simulink model "simulation_darko_complet_fuel_op"  (R2020b)
settings: Solver=VariableStepAuto  StartTime=0.0  StopTime=20  RelTol=1e-3
values from neighbouring files (symbols this model uses):
  controlleur = generateContolleur(drone)    [run_darko_droit_complet_fuel_op.m]
  drone = struct('MASS',               0.492,                      'INERTIA',            eye(3),                     'G',                  9.81,                       'P_P1_CG',            [1; 1; 1],                  'P_P2_CG',            [1; 1; 1],                  'P_A1_CG',            [1; 1; 1],                  'P_A2_CG',            [1; 1; 1],                  'INERTIA_PROP_X',     5.1116e-6,            ...(+959 chars)    [generateDarko.m]    (also in run_darko_droit_complet_fuel_op.m = generateDarko())
  f_initial = drone.MASS*drone.G    [run_darko_droit_complet_fuel_op.m]
  initial_state = [p_initial; v_initial; omega_initial; q_initial]    [run_darko_droit_complet_fuel_op.m]
  position_cible = 1*[1; 1; 1]    [run_darko_droit_complet_fuel_op.m]
  q_d_initial = ToQuaternion(yaw_d, pitch_d, roll_d)    [run_darko_droit_complet_fuel_op.m]
libraries: simulink_extras x3, sharedtransform x1
settings Model: Creator=florian  LastModifiedBy=florian

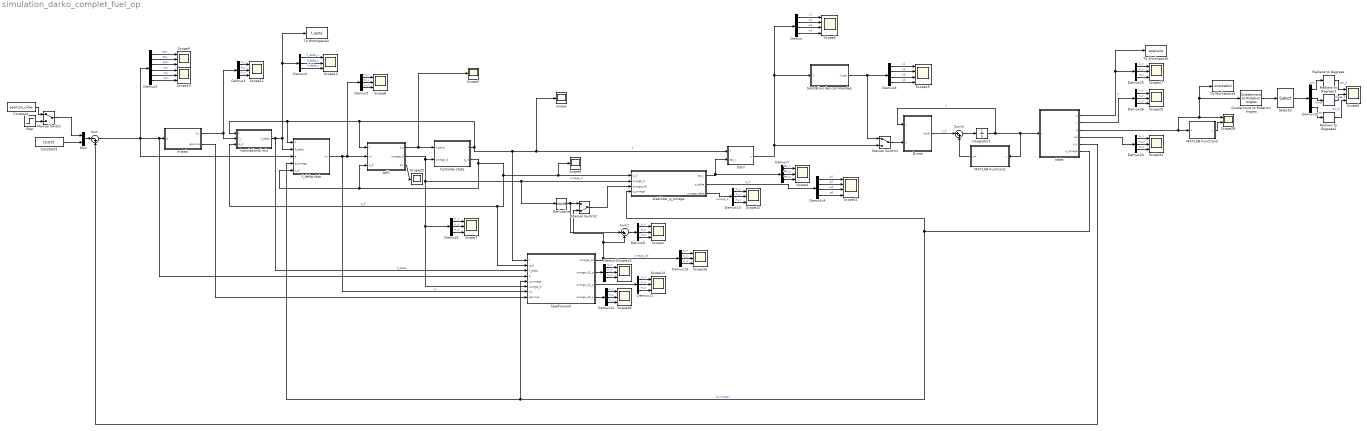
== system simulation_darko_complet_fuel_op ==
  Constant : Constant  Value=position_cible
  Constant1 : Constant  Value=[0;0;0]
  Contoller state : Subsystem
  Demux : Demux
  Demux{1,3..7,9..13,15,24..26} (15 alike) : Demux  Outputs=3
  Demux14 : Demux
  Demux2 : Demux  Outputs=6
  Demux8 : Demux
  Derivative : Derivative  CoefficientInTFapproximation=1/1000
  Drone : MATLAB Function  TreatAsAtomicUnit=on
  Integrator1 : Integrator  InitialCondition=initial_state
  MATLAB Function2 : MATLAB Function  TreatAsAtomicUnit=on
  MATLAB Function3 : MATLAB Function  TreatAsAtomicUnit=on
  Manual Switch : ManualSwitch
  Manual Switch1 : ManualSwitch
  Manual Switch2 : ManualSwitch  CurrentSetting=0
  Mux : Mux  Inputs=2
  Quaternions to Rotation Angles : sharedtransform/Quaternions to Rotation Angles  rotationOrder=ZXY  aMode=aMode
      settings: SourceProductBaseCode=AE,PW,MT,UV,VE,VP
  Radians to Degrees : simulink_extras/Transformations/Radians to Degrees
  Radians to Degrees1 : simulink_extras/Transformations/Radians to Degrees
  Radians to Degrees2 : simulink_extras/Transformations/Radians to Degrees
  Satutation des commandes : Subsystem
  Scope{,2,6,20} (4 alike) : Scope
  Scope{1,3..4,7..14,16,18,22,27,29,34} (17 alike) : Scope  NumInputPorts=3
  Scope15 : Scope  NumInputPorts=4
  Scope21 : Scope  NumInputPorts=4
  Scope28 : Scope  NumInputPorts=2
  Scope5 : Scope  NumInputPorts=4
  Selector : Selector  InputPortWidth=3  IndexOptions=Index vector (dialog)  Indices=[2 3 1]  OutputSizes=1
  Step : Step  Time=10  Before=position_cible  After=[0;0;0]  SampleTime=0
  Sum : Sum  Inputs=|-+
  Sum1 : Sum  Inputs=|+-
  Sum5 : Sum  Inputs=|++
  To Workspace1 : ToWorkspace  VariableName=positions  SampleTime=-1
  To Workspace2 : ToWorkspace  VariableName=f_delta  SampleTime=-1
  To Workspace3 : ToWorkspace  VariableName=orientation  SampleTime=-1
  distri : MATLAB Function  TreatAsAtomicUnit=on
  e stab : MATLAB Function  TreatAsAtomicUnit=on
  f_delta stab : MATLAB Function  TreatAsAtomicUnit=on
  feedforward : MATLAB Function  TreatAsAtomicUnit=on
  split : MATLAB Function  TreatAsAtomicUnit=on
  stabilizer_q_omega : MATLAB Function  TreatAsAtomicUnit=on
  state : MATLAB Function  TreatAsAtomicUnit=on
  translational mis : MATLAB Function  TreatAsAtomicUnit=on
  wires:
  Manual Switch/1 -> Mux/1
  Mux/1 -> Sum/1
  f_delta stab/1(nu) -> feedforward/7(nu), Demux5/1, split/2(nu)  "nu"
  Demux4/2 -> Scope12/2  "f_delta_y"
  Contoller state/2(q_d) -> f_delta stab/5(q_d), split/3(q_d), feedforward/2(q_d), translational mis/3(q_d), Scope6/1, stabilizer_q_omega/1(q_d)  "q_d"
  Step/1 -> Manual Switch/2
  Demux9/2 -> Scope7/2  "w_y"
  Demux2/4 -> Scope10/1  "vpx"
  stabilizer_q_omega/3(omega_delta) -> Demux15/1  "omega_d"
  Demux15/3 -> Scope22/3  "w_z"
  split/2(omega_d) -> feedforward/6(omega_d), Demux9/1, Derivative/1, stabilizer_q_omega/2(omega_d), Contoller state/2(omega_d)  "omega_d"
  translational mis/1(f_delta) -> feedforward/3(f_delta), Demux4/1, To Workspace2/1, f_delta stab/2(f_delta)  "f_delta"
  Demux15/1 -> Scope22/1  "w_x"
  Demux15/2 -> Scope22/2  "w_y"
  Demux2/1 -> Scope9/1  "epx"
  Demux2/5 -> Scope10/2  "vpy"
  Constant/1 -> Manual Switch/1
  Demux3/3 -> Scope11/3  "fr_z"
  Demux4/3 -> Scope12/3  "f_delta_z"
  Constant1/1 -> Mux/2
  Demux5/1 -> Scope8/1  "nu_x"
  Demux4/1 -> Scope12/1  "f_delta_x"
  stabilizer_q_omega/1(tau_r) -> Demux7/1, distri/2(tau_r)
  split/1(f_d) -> Scope2/1, Contoller state/1(f_point)
  Demux5/3 -> Scope8/3  "nu_z"
  Demux9/3 -> Scope7/3  "w_z"
  split/3(err) -> Scope20/1
  Demux3/1 -> Scope11/1  "fr_x"
  Contoller state/1(f) -> f_delta stab/1(f), translational mis/1(f), split/1(f), feedforward/1(f), Scope/1, distri/1(f)  "f"
  Demux2/6 -> Scope10/3  "vpz"
  Demux3/2 -> Scope11/2  "fr_y"
  Demux2/2 -> Scope9/2  "epy"
  Demux9/1 -> Scope7/1  "w_x"
  Demux2/3 -> Scope9/3  "epz"
  Demux5/2 -> Scope8/2  "nu_y"
  e stab/1(f_r) -> translational mis/2(f_r), Demux3/1
  Sum/1 -> feedforward/4(e), e stab/1(e), f_delta stab/3(e), Demux2/1
  Manual Switch2/1 -> stabilizer_q_omega/3(omega_dd)
  Derivative/1 -> Sum1/1, Manual Switch2/1
  feedforward/1(omega_dd) -> Demux13/1, Sum1/2, Manual Switch2/2  "omega_dd"
  Demux1/3 -> Scope13/3  "w_z"
  feedforward/4(omega_d3_p) -> Demux12/1
  Demux11/2 -> Scope14/2  "w_y"
  Demux12/3 -> Scope18/3  "w_z"
  feedforward/2(omega_d1_p) -> Demux1/1
  Demux12/1 -> Scope18/1  "w_x"
  Demux11/1 -> Scope14/1  "w_x"
  Demux1/2 -> Scope13/2  "w_y"
  Demux11/3 -> Scope14/3  "w_z"
  Demux12/2 -> Scope18/2  "w_y"
  feedforward/3(omega_d2_p) -> Demux11/1
  Demux1/1 -> Scope13/1  "w_x"
  e stab/2(gamma) -> feedforward/8(gamma)
  Demux7/2 -> Scope4/2  "tau_y"
  Satutation des commandes/1(U_sat) -> Manual Switch1/1, Demux8/1
  state/2(v) -> Demux26/1
  Demux25/1 -> Scope27/1  "p_x"
  Demux26/1 -> Scope29/1  "v_x"
  Integrator1/1 -> Drone/1(x), MATLAB Function2/1(x), state/1(x)  "x"
  state/1(p) -> To Workspace1/1, Demux25/1  "p"
  Demux/1 -> Scope5/1  "u1"
  distri/1(u) -> Satutation des commandes/1(U), Demux/1, Manual Switch1/2
  Sum5/1 -> Integrator1/1
  state/3(q) -> Scope28/1, To Workspace3/1, Quaternions to Rotation Angles/1, MATLAB Function3/1(u)
  Demux24/1 -> Scope34/1  "w_x"
  Demux25/2 -> Scope27/2  "p_y"
  Demux7/3 -> Scope4/3  "tau_z"
  Demux/2 -> Scope5/2  "u2"
  stabilizer_q_omega/2(q_delta) -> Demux14/1  "q_d"
  Drone/1(dxdt) -> Sum5/1  "x_d"
  Demux8/2 -> Scope15/2  "u2"
  MATLAB Function3/1(y) -> Scope28/2
  Demux7/1 -> Scope4/1  "tau_x"
  Demux14/3 -> Scope21/3  "q3"
  state/6(q_omega) -> stabilizer_q_omega/4(q_omega), feedforward/5(q_omega), f_delta stab/4(q_omega)  "(q,omega)"
  Demux25/3 -> Scope27/3  "p_z"
  MATLAB Function2/1(cor) -> Sum5/2
  Manual Switch1/1 -> Drone/2(u)
  Demux14/4 -> Scope21/4  "q4"
  Demux26/3 -> Scope29/3  "v_z"
  Demux8/4 -> Scope15/4  "u4"
  Demux8/1 -> Scope15/1  "u1"
  Demux14/1 -> Scope21/1  "q1"
  Demux/4 -> Scope5/4  "u4"
  Demux24/3 -> Scope34/3  "w_z"
  Demux14/2 -> Scope21/2  "q2"
  Demux8/3 -> Scope15/3  "u3"
  state/5(p_v) -> Sum/2
  state/4(wb) -> Demux24/1
  Demux/3 -> Scope5/3  "u3"
  Demux24/2 -> Scope34/2  "w_y"
  Demux26/2 -> Scope29/2  "v_y"
  Quaternions to Rotation Angles/1 -> Selector/1
  Radians to Degrees1/1 -> Scope3/2  "theta_d"
  Demux10/1 -> Radians to Degrees/1  "phi"
  Demux10/3 -> Radians to Degrees2/1  "psi"
  Selector/1 -> Demux10/1
  Radians to Degrees/1 -> Scope3/1  "phi_d"
  Demux10/2 -> Radians to Degrees1/1  "theta"
  Radians to Degrees2/1 -> Scope3/3  "psi_d"
  Sum1/1 -> Demux6/1
  Demux6/1 -> Scope1/1  "w_x"
  Demux6/3 -> Scope1/3  "w_z"
  Demux6/2 -> Scope1/2  "w_y"
  Demux13/1 -> Scope16/1  "w_x"
  Demux13/3 -> Scope16/3  "w_z"
  Demux13/2 -> Scope16/2  "w_y"

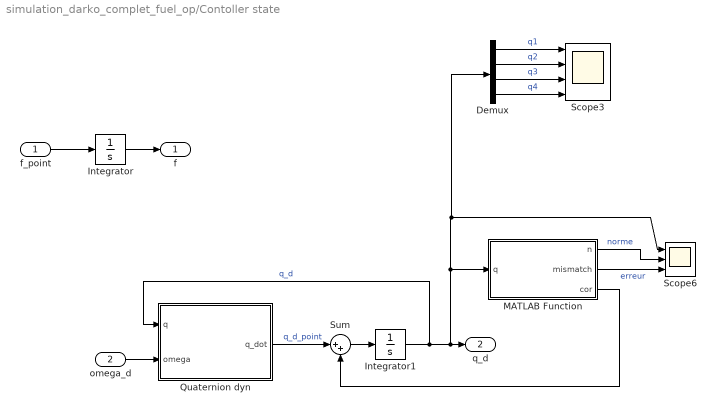
== system simulation_darko_complet_fuel_op/Contoller state ==
  f_point : Inport
  omega_d : Inport  Port=2
  Demux : Demux
  Integrator : Integrator  InitialCondition=f_initial
  Integrator1 : Integrator  InitialCondition=q_d_initial
  MATLAB Function : MATLAB Function  TreatAsAtomicUnit=on
  Quaternion dyn : MATLAB Function  TreatAsAtomicUnit=on
  Scope3 : Scope  NumInputPorts=4
  Scope6 : Scope  NumInputPorts=3
  Sum : Sum  Inputs=|++
  f : Outport
  q_d : Outport  Port=2
  wires:
  Integrator/1 -> f/1
  f_point/1 -> Integrator/1
  Integrator1/1 -> Quaternion dyn/1(q), Demux/1, Scope6/1, MATLAB Function/1(q), q_d/1  "q_d"
  omega_d/1 -> Quaternion dyn/2(omega)
  Quaternion dyn/1(q_dot) -> Sum/1  "q_d_point"
  Sum/1 -> Integrator1/1
  MATLAB Function/3(cor) -> Sum/2
  MATLAB Function/1(n) -> Scope6/2  "norme"
  MATLAB Function/2(mismatch) -> Scope6/3  "erreur"
  Demux/3 -> Scope3/3  "q3"
  Demux/2 -> Scope3/2  "q2"
  Demux/1 -> Scope3/1  "q1"
  Demux/4 -> Scope3/4  "q4"

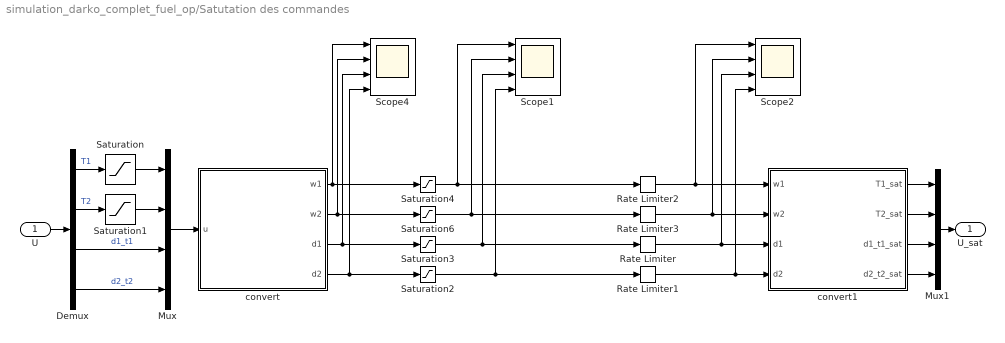
== system simulation_darko_complet_fuel_op/Satutation des commandes ==
  U : Inport
  Demux : Demux
  Mux : Mux
  Mux1 : Mux
  Rate Limiter : RateLimiter  RisingSlewLimit=drone.ELEVON_RATE_CHANGE  FallingSlewLimit=-drone.ELEVON_RATE_CHANGE  SampleTimeMode=inherited
  Rate Limiter1 : RateLimiter  RisingSlewLimit=drone.ELEVON_RATE_CHANGE  FallingSlewLimit=-drone.ELEVON_RATE_CHANGE  SampleTimeMode=inherited
  Rate Limiter2 : RateLimiter  RisingSlewLimit=drone.MOTOR_RATE_CHANGE  FallingSlewLimit=-drone.MOTOR_RATE_CHANGE  SampleTimeMode=inherited
  Rate Limiter3 : RateLimiter  RisingSlewLimit=drone.MOTOR_RATE_CHANGE  FallingSlewLimit=-drone.MOTOR_RATE_CHANGE  SampleTimeMode=inherited
  Saturation : Saturate  UpperLimit=100  LowerLimit=0.001
  Saturation1 : Saturate  UpperLimit=100  LowerLimit=0.001
  Saturation2 : Saturate  UpperLimit=30*(pi/180)  LowerLimit=-30*(pi/180)
  Saturation3 : Saturate  UpperLimit=30*(pi/180)  LowerLimit=-30*(pi/180)
  Saturation4 : Saturate  UpperLimit=1000  LowerLimit=200
  Saturation6 : Saturate  UpperLimit=1000  LowerLimit=200
  Scope1 : Scope  NumInputPorts=4
  Scope2 : Scope  NumInputPorts=4
  Scope4 : Scope  NumInputPorts=4
  convert : MATLAB Function  TreatAsAtomicUnit=on
  convert1 : MATLAB Function  TreatAsAtomicUnit=on
  U_sat : Outport
  wires:
  U/1 -> Demux/1
  Demux/4 -> Mux/4  "d2_t2"
  Demux/1 -> Saturation/1  "T1"
  Demux/3 -> Mux/3  "d1_t1"
  Demux/2 -> Saturation1/1  "T2"
  Saturation/1 -> Mux/1
  Mux/1 -> convert/1(u)
  convert/1(w1) -> Saturation4/1, Scope4/1
  Saturation3/1 -> Rate Limiter/1, Scope1/3
  convert/2(w2) -> Scope4/2, Saturation6/1
  convert/3(d1) -> Scope4/3, Saturation3/1
  convert/4(d2) -> Saturation2/1, Scope4/4
  convert1/1(T1_sat) -> Mux1/1
  convert1/4(d2_t2_sat) -> Mux1/4
  Mux1/1 -> U_sat/1
  Saturation1/1 -> Mux/2
  convert1/2(T2_sat) -> Mux1/2
  convert1/3(d1_t1_sat) -> Mux1/3
  Saturation2/1 -> Rate Limiter1/1, Scope1/4
  Rate Limiter/1 -> Scope2/3, convert1/3(d1)
  Saturation6/1 -> Rate Limiter3/1, Scope1/2
  Saturation4/1 -> Rate Limiter2/1, Scope1/1
  Rate Limiter1/1 -> Scope2/4, convert1/4(d2)
  Rate Limiter2/1 -> Scope2/1, convert1/1(w1)
  Rate Limiter3/1 -> Scope2/2, convert1/2(w2)

== matlab function simulation_darko_complet_fuel_op/feedforward ==
  data: f input; omega_dd output; q_d input; f_delta input; e input; q_omega input; omega_d input; nu input; gamma input; controlleur parameter; drone parameter; omega_d1_p output; omega_d2_p output; omega_d3_p output
function [omega_dd, omega_d1_p, omega_d2_p, omega_d3_p]  = feedforward(f, q_d, f_delta, e, q_omega, omega_d, nu, gamma, controlleur, drone)
%#codegen

d_etoile = controlleur.d_etoile;
kpp = controlleur.kpp;
kpd = controlleur.kpd;
k_delta = controlleur.k_delta;
m = drone.MASS;

a = controlleur.a;
b = controlleur.b;
c = controlleur.c;

ep = e(1:3);
ev = e(4:6);

q = q_omega(1:4);
omega = q_omega(5:7);

R = q2dcm(q);
Rd = q2dcm(q_d);

omega_d1_p = -(1/(f^2)) * skew_sym(d_etoile) * Rd' * nu * ( Rd * d_etoile)' * nu;
omega_d2_p = -(1/(f))* skew_sym(d_etoile) * skew_sym(omega_d) * Rd' * nu;

% ev_dot = 1/m*((R-Rd)*d_etoile*f - gamma + f_delta);
% 
% u = kpp*(ep + ev.*sqrt((abs(ev)/(2*a)).^2 + (kpd/kpp)^2));
% u_dot = kpp*(ev + ev_dot .* sqrt((abs(ev)/(2*a)).^2 + (kpd/kpp)^2) + ev .* abs(ev)./(2*a*sqrt((abs(ev)/(2*a)).^2 + (kpd/kpp)^2)));
% 
% gamma_dot = 2*a*b*c*u_dot.*exp(-c*u).*exp(-b*exp(-c*u));
% f_delta_dot = nu - gamma_dot;
% 
% term_1 = (kpp*kpd/m)*ev;
% term_2 = (kpd^2/m^2 - kpp/m) * ev_dot;
% term_3 = -(kpd/m + k_delta)*f_delta_dot;
% 
% omega_d3_p = (1/f) * skew_sym(d_etoile) * Rd'* (term_1 + term_2 + term_3); 

Gain = (kpd^2/m^2 - kpp/m);

ep_term = - Gain*kpp*ep;
ev_term = (kpp*kpd/m - Gain*kpd)*ev;
f_delta_term = (Gain + (kpd/m + k_delta)*k_delta)*f_delta;
f_term = (Gain*(R-Rd) + kpd/m * (Rd*skew_sym(omega_d) - R*skew_sym(omega)))*d_etoile* f;
nu_term = kpd/m * (Rd-R) * d_etoile * (Rd*d_etoile)'* nu;

omega_d3_p = (1/f) * skew_sym(d_etoile) * Rd'* (ep_term + ev_term + f_delta_term + f_term + nu_term); 


omega_dd = omega_d1_p + omega_d2_p + omega_d3_p ; %

== matlab function simulation_darko_complet_fuel_op/Contoller state/MATLAB Function ==
  data: n output; q input; mismatch output; cor output
function [n, mismatch, cor] = fcn(q)
%#codegen
n = norm(q);
mismatch = 1-norm(q);
cor = mismatch*q;

== matlab function simulation_darko_complet_fuel_op/Satutation des commandes/convert ==
  data: u input; w1 output; drone parameter; w2 output; d1 output; d2 output
function [w1, w2, d1, d2] = convert(u, drone)
%#codegen
kf = drone.PROP_KP;

T1 = max(u(1), 0);
T2 = max(u(2), 0);
% T1 = u(1);
% T2 = u(2);

d1_T1 = u(3);
d2_T2 = u(4);

w1 = sqrt(T1/kf);
w2 = sqrt(T2/kf);
d1 = d1_T1/T1;
d2 = d2_T2/T2;

== matlab function simulation_darko_complet_fuel_op/Contoller state/Quaternion dyn ==
  data: q input; q_dot output; omega input
function q_dot = q_dyn(q, omega)
%#codegen

eta = q(1);
eps = q(2:4);

A = [-eps';  eta*eye(3)+skew_sym(eps)];
q_dot = 1/2*A*omega;

== matlab function simulation_darko_complet_fuel_op/Satutation des commandes/convert1 ==
  data: w1 input; w2 input; d1 input; d2 input; T1_sat output; T2_sat output; drone parameter; d1_t1_sat output; d2_t2_sat output
function [T1_sat, T2_sat, d1_t1_sat, d2_t2_sat] = convert2(w1, w2, d1, d2, drone)
%#codegen
kf = drone.PROP_KP;

T1_sat = kf*w1^2;
d1_t1_sat = d1*T1_sat;
T2_sat = kf*w2^2;
d2_t2_sat = d2*T2_sat;

== matlab function simulation_darko_complet_fuel_op/MATLAB Function2 ==
  data: x input; cor output
function cor  = fcn(x)
%#codegen
q  = x(7:10);
n = norm(q);
mismatch = 1-n;
cor = [0;0;0; 0;0;0; mismatch*q; 0;0;0];

== matlab function simulation_darko_complet_fuel_op/MATLAB Function3 ==
  data: u input; y output
function y = fcn(u)
%#codegen

y = norm(u);

== matlab function simulation_darko_complet_fuel_op/state ==
  data: x input; p output; v output; q output; wb output; p_v output; q_omega output
function [p, v,q, wb, p_v, q_omega] = demux(x)
%#codegen

p = x(1:3);
v = x(4:6);
q  = x(7:10);
wb = x(11:13);

p_v = x(1:6);
q_omega = x(7:13);

== matlab function simulation_darko_complet_fuel_op/distri ==
  data: f input; u output; tau_r input; controlleur parameter
function u = dist(f,tau_r, controlleur)
%#codegen
u = controlleur.M_k * tau_r + controlleur.u_barre * f;

== matlab function simulation_darko_complet_fuel_op/Drone ==
  data: x input; u input; dxdt output; drone parameter
function dxdt = drone(x, u, drone)

%% physical constants
% gravity
g = drone.G;
% vehicle mass
m = drone.MASS;
% vehicle inertia matrix
J = drone.INERTIA; % [3x3 real symmetric] in body axis

%% state demultiplexing
% p = x(1:3);
v = x(4:6);
q  = x(7:10);
wb = x(11:13);

Rq = q2dcm(q);

[Fp, Mp] = external_force_moment(x, u, 0, drone);

% position
dpdt = v;

% kinematics
dvdt =  -[0;0;g] + (1/m)*Rq*drone.Fb*u + (1/m)*Rq*Fp; 


%% quaternion derivative
eta = q(1);
eps = q(2:4);

dqdt = (1/2)*[-eps'; eta*eye(3) + skew_sym(eps)]*wb;

%% angular velocity derivative
% kinematics
dwdt = -J\cross(wb, J*wb) + J\(drone.Mb*u) + J\Mp;

%% derivative multiplexing
dxdt = [dpdt; dvdt; dqdt; dwdt] ;

== matlab function simulation_darko_complet_fuel_op/stabilizer_q_omega ==
  data: q_d input; omega_d input; omega_dd input; q_omega input; tau_r output; controlleur parameter; drone parameter; q_delta output; omega_delta output
function [tau_r, q_delta, omega_delta]  = stabilizer_q_omega(q_d, omega_d, omega_dd, q_omega, controlleur, drone )

J = drone.INERTIA;

q = q_omega(1:4);
omega = q_omega(5:7);

eta = q(1);
eps = q(2:4);

eta_d = q_d(1);
eps_d = q_d(2:4);

eta_delta = eta_d*eta + eps_d'*eps;
eps_delta = -eta*eps_d + eta_d*eps - skew_sym(eps_d)*eps;

omega_delta = omega - omega_d;

tau_r = - controlleur.kap * eps_delta - controlleur.kad * omega_delta + cross(omega, J* omega) + J*omega_dd;
q_delta = [eta_delta; eps_delta];
end

== matlab function simulation_darko_complet_fuel_op/split ==
  data: f input; nu input; f_d output size=1; q_d input; omega_d output size=3; controlleur parameter; err output
function [f_d, omega_d, err] = split(f, nu, q_d, controlleur)
%#codegen

R_d = q2dcm(q_d);

f_d = (R_d * controlleur.d_etoile)' * nu;
omega_d = 1/f * controlleur.skew_sym_d_etoile * R_d' * nu;

err =  R_d*controlleur.d_etoile*f_d + R_d* skew_sym(omega_d) * controlleur.d_etoile * f - nu;

== matlab function simulation_darko_complet_fuel_op/f_delta stab ==
  data: f input; f_delta input; nu output; e input; q_omega input; q_d input; controlleur parameter; drone parameter
function nu = stab_f_delta(f, f_delta, e, q_omega, q_d, controlleur, drone)
%#codegen
m = drone.MASS;
kpp = controlleur.kpp;
kpd = controlleur.kpd;
k_delta = controlleur.k_delta;

ep = e(1:3);
ev = e(4:6);

q = q_omega(1:4);
% omega = q_omega(5:7);

R = q2dcm(q);
Rd = q2dcm(q_d);

nu = ((kpp * kpd)/m) * ep + (kpd^2/m - kpp) * ev - (kpd/m + k_delta) * f_delta -kpd/m * (R-Rd) * controlleur.d_etoile * f;

== matlab function simulation_darko_complet_fuel_op/translational mis ==
  data: f input; f_r input; f_delta output; q_d input; controlleur parameter
function f_delta = trans_mis(f, f_r,  q_d, controlleur)
%#codegen

f_delta = q2dcm(q_d) * controlleur.d_etoile * f - f_r;

== matlab function simulation_darko_complet_fuel_op/e stab ==
  data: e input; f_r output; drone parameter; controlleur parameter; gamma output
function [f_r, gamma] = e_stab(e, drone, controlleur)
    
    b = controlleur.b;
    c = controlleur.c;
    sat = @(x) 2*controlleur.a*exp(-b*exp(-c*x)) -controlleur.a;
    
    ep = e(1:3);
    ev = e(4:6);
    QTO = sat(controlleur.kpp * (ep + ev .* nthroot((abs(ev)/(2*controlleur.a)).^4 + (controlleur.kpd/controlleur.kpp)^4, 4)));

%     f_r = drone.MASS * [0;0;drone.G] - controlleur.kpp * ep - controlleur.kpd * ev;
    f_r = drone.MASS * [0;0;drone.G] - QTO;
    gamma = QTO;
end
